simulink model "processo_tanque_2"  (R2017b)
settings: Solver=VariableStepAuto  StartTime=0.0  StopTime=120.0  RelTol=1e-3
settings Model: Creator=fernandopassold  LastModifiedBy=fernandopassold
settings CodeAppCC: StateflowObjectComments=on

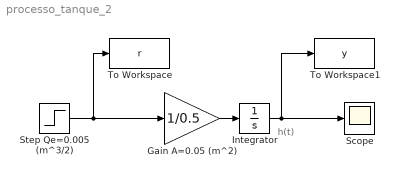
== system processo_tanque_2 ==
  note: h(t)
  Gain A=0.05 (m^2) : Gain  Gain=1/0.5
  Integrator : Integrator
  Scope : Scope
  Step Qe=0.005 (m^3/2) : Step  Time=10  After=0.005  SampleTime=0
  To Workspace : ToWorkspace  VariableName=r  SaveFormat=Timeseries  SampleTime=-1
  To Workspace1 : ToWorkspace  VariableName=y  SaveFormat=Timeseries  SampleTime=-1
  wires:
  Gain A=0.05 (m^2)/1 -> Integrator/1
  Integrator/1 -> To Workspace1/1, Scope/1
  Step Qe=0.005 (m^3/2)/1 -> To Workspace/1, Gain A=0.05 (m^2)/1
